simulink model "Problem7"  (R2020b)
settings: Solver=VariableStepAuto  StartTime=0.0  StopTime=10.0  RelTol=1e-3
settings Model: Creator=Dell  LastModifiedBy=Dell

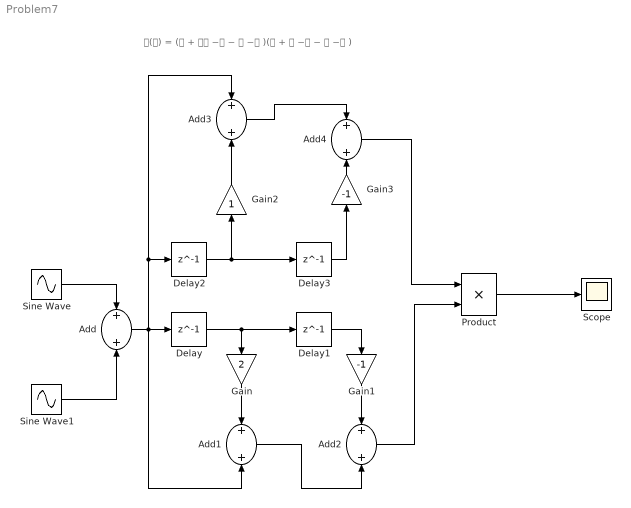
== system Problem7 ==
  note: 𝐇(𝐳) = (𝟏 + 𝟐𝐳 −𝟏 − 𝐳 −𝟐 )(𝟏 + 𝐳 −𝟏 − 𝐳 −𝟐 )
  Add{,1..4} (5 alike) : Sum
  Delay{,1..3} (4 alike) : Delay  DelayLength=1
  Gain : Gain  Gain=2
  Gain1 : Gain  Gain=-1
  Gain2 : Gain
  Gain3 : Gain  Gain=-1
  Product : Product
  Scope : Scope
  Sine Wave : Sin  SampleTime=0
  Sine Wave1 : Sin  SampleTime=0
  wires:
  Sine Wave/1 -> Add/1
  Sine Wave1/1 -> Add/2
  Gain/1 -> Add1/1
  Add/1 -> Delay2/1, Add3/1, Add1/2, Delay/1
  Delay/1 -> Delay1/1, Gain/1
  Gain1/1 -> Add2/1
  Add1/1 -> Add2/2
  Delay1/1 -> Gain1/1
  Add2/1 -> Product/2
  Delay2/1 -> Delay3/1, Gain2/1
  Delay3/1 -> Gain3/1
  Add3/1 -> Add4/1
  Gain3/1 -> Add4/2
  Gain2/1 -> Add3/2
  Add4/1 -> Product/1
  Product/1 -> Scope/1
